simulink model "Stand_AOPO"  (R2018b)
settings: Solver=FixedStepAuto  StartTime=0.0  StopTime=inf  FixedStep=1e-3  RelTol=1e-3
libraries: simulink x17, simulink_extras x4, xpcutilitieslib x2, xpcrtudplib x2, opclib x1, sldrtlib x1
settings Model: Creator=YuORLOV  LastModifiedBy=9
settings DataIOCC: SaveTime=off
settings OptimizationCC: BlockReduction=off
settings DebuggingCC: LibraryContextMissingDiagnostic=none
settings SFSimCC: SimUseLocalCustomCode=off
settings RTWCC: RTWUseLocalCustomCode=off
settings CodeAppCC: StateflowObjectComments=on
settings SimscapeCC: SimscapeNormalizeSystem=off

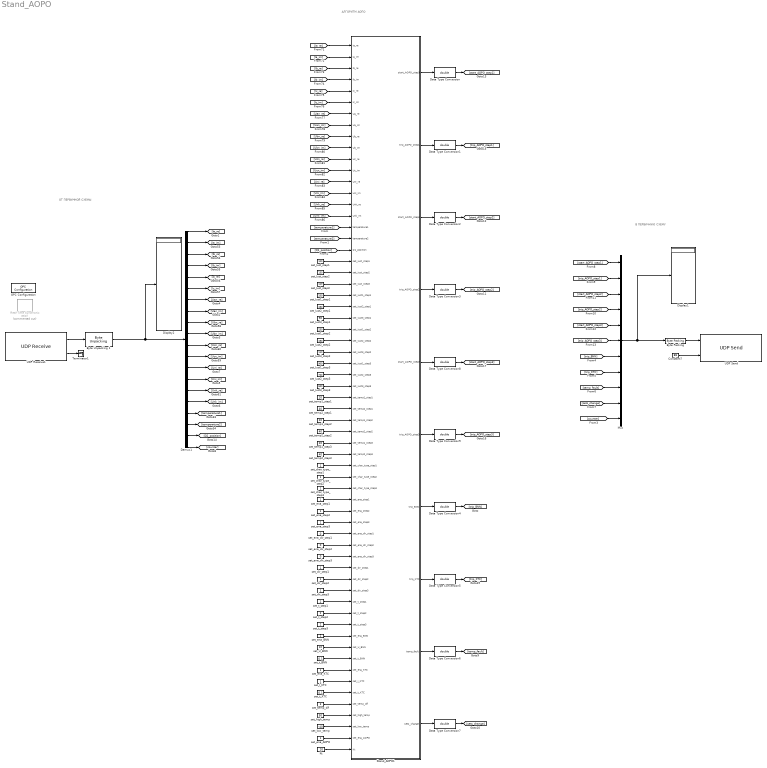
== system Stand_AOPO ==
  note: ОТ ПЕРВИЧНОЙ СХЕМЫ
  note: АЛГОРИТМ АОПО
  note: В ПЕРВИЧНУЮ СХЕМУ
  "Byte Packing " : xpcutilitieslib/Byte Packing   MaskPackedDataType=uint8  MaskUnpackedDataTypes={'double'}  MaskAlignment=1
  Byte Unpacking 1 : xpcutilitieslib/Byte Unpacking   MaskUnpackedDataTypes={'double'}  MaskUnpackedDataSizes={[20]}  MaskAlignment=1
      settings: SourceProductName=Simulink Real-Time  SourceProductBaseCode=XP
  Constant7 : Constant  Value=88
  Data Type Conversion{,1..9} (10 alike) : DataTypeConversion  OutDataTypeStr=double
  Demux1 : Demux  Outputs=20
  Display1 : Display
  Display2 : Display
  Kt : Constant  Value=20
  Mux : Mux  Inputs=11
  OPC Configuration : opclib/OPC Configuration  errMissingItems=Error  errReadWrite=Warn  errShutdown=Error  errRTViolation=Warn  rtEnable=on  speedup=1  showLatency=off  beingUsed=on
      settings: SourceProductName=OPC Toolbox  SourceProductBaseCode=OT
  Real-Time Synchronization : sldrtlib/Real-Time Synchronization  Commented=on  SampleTime=0.1  MaxMissedTicks=10  ShowMissedTicks=off  YieldWhenWaiting=off
  Stand_AOPO1 : Subsystem
  Terminator1 : Terminator
  UDP Receive1 : xpcrtudplib/UDP Receive  ipAddressVal=Use host-target connection  localPort=25001  rcvWidth=160  rcvFmAny=off  fmAddress=192.168.1.251  rcvMulticast=off  multicastAddress=[]  maxUDPQueue=8  sampleTime=1e-3
      settings: SourceProductName=Simulink Real-Time
  UDP Send : xpcrtudplib/UDP Send  ipAddressVal=Use host-target connection  localPort=25002  toAddress=192.168.1.251  toPort=8002  sampleTime=1e-3
      settings: SourceProductName=Simulink Real-Time  SourceProductBaseCode=XP
  set_I_KTC : Constant
  set_Iust1_step1 : Constant  Value=200
  set_Iust1_step2 : Constant  Value=250
  set_Iust1_step3 : Constant  Value=900
  set_Iust2_step1 : Constant  Value=160
  set_Iust2_step2 : Constant  Value=190
  set_Iust2_step3 : Constant  Value=700
  set_Iust3_step1 : Constant  Value=90
  set_Iust3_step2 : Constant  Value=110
  set_Iust3_step3 : Constant  Value=500
  set_Iust_step1 : Constant  Value=120
  set_Iust_step2 : Constant  Value=130
  set_Iust_step3 : Constant  Value=140
  set_U_BNN : Constant  Value=10
  set_char_type_step1 : Constant
  set_char_type_step2 : Constant
  set_char_type_step3 : Constant
  set_dir_step1 : Constant
  set_dir_step2 : Constant
  set_dir_step3 : Constant
  set_ena_AOPO : Constant
  set_ena_BNN : Constant
  set_ena_KTC : Constant
  set_ena_dir_step1 : Constant  Value=0
  set_ena_dir_step2 : Constant  Value=0
  set_ena_dir_step3 : Constant  Value=0
  set_ena_step1 : Constant
  set_ena_step2 : Constant
  set_ena_step3 : Constant
  set_high_temp : Constant  Value=50
  set_low_temp : Constant  Value=-40
  set_t_BNN : Constant  Value=0.1
  set_t_KTC : Constant  Value=0.1
  set_t_step1 : Constant  Value=2
  set_t_step2 : Constant  Value=2
  set_t_step3 : Constant  Value=2
  set_temp1_step1 : Constant  Value=20
  set_temp1_step2 : Constant  Value=20
  set_temp1_step3 : Constant  Value=20
  set_temp2_step1 : Constant  Value=40
  set_temp2_step2 : Constant  Value=40
  set_temp2_step3 : Constant  Value=40
  set_temp_dif : Constant  Value=3
  wires:
  Mux/1 -> Display1/1, "Byte Packing "/1
  Constant7/1 -> UDP Send/2
  "Byte Packing "/1 -> UDP Send/1
  set_Iust_step1/1 -> Stand_AOPO1/20(set_Iust_step1)
  set_Iust_step2/1 -> Stand_AOPO1/21(set_Iust_step2)
  set_U_BNN/1 -> Stand_AOPO1/54(set_U_BNN)
  set_t_step1/1 -> Stand_AOPO1/50(set_t_step1)
  set_t_step2/1 -> Stand_AOPO1/51(set_t_step2)
  set_t_BNN/1 -> Stand_AOPO1/55(set_t_BNN)
  set_I_KTC/1 -> Stand_AOPO1/57(set_I_KTC)
  set_t_KTC/1 -> Stand_AOPO1/58(set_t_KTC)
  set_ena_step1/1 -> Stand_AOPO1/41(set_ena_step1)
  set_ena_step2/1 -> Stand_AOPO1/42(set_ena_step2)
  set_ena_AOPO/1 -> Stand_AOPO1/62(set_ena_AOPO)
  set_ena_KTC/1 -> Stand_AOPO1/56(set_ena_KTC)
  set_dir_step2/1 -> Stand_AOPO1/48(set_dir_step2)
  set_dir_step1/1 -> Stand_AOPO1/47(set_dir_step1)
  set_ena_dir_step2/1 -> Stand_AOPO1/45(set_ena_dir_step2)
  set_ena_dir_step1/1 -> Stand_AOPO1/44(set_ena_dir_step1)
  set_ena_BNN/1 -> Stand_AOPO1/53(set_ena_BNN)
  set_char_type_step2/1 -> Stand_AOPO1/39(set_char_type_step2)
  set_char_type_step1/1 -> Stand_AOPO1/38(set_char_type_step1)
  set_temp2_step2/1 -> Stand_AOPO1/35(set_temp2_step2)
  set_temp1_step2/1 -> Stand_AOPO1/34(set_temp1_step2)
  set_temp2_step1/1 -> Stand_AOPO1/33(set_temp2_step1)
  set_temp1_step1/1 -> Stand_AOPO1/32(set_temp1_step1)
  set_Iust3_step2/1 -> Stand_AOPO1/28(set_Iust3_step2)
  set_Iust2_step2/1 -> Stand_AOPO1/27(set_Iust2_step2)
  set_Iust1_step2/1 -> Stand_AOPO1/26(set_Iust1_step2)
  set_Iust3_step1/1 -> Stand_AOPO1/25(set_Iust3_step1)
  set_Iust2_step1/1 -> Stand_AOPO1/24(set_Iust2_step1)
  set_Iust1_step1/1 -> Stand_AOPO1/23(set_Iust1_step1)
  Byte Unpacking 1/1 -> Demux1/1, Display2/1
  UDP Receive1/1 -> Byte Unpacking 1/1
  UDP Receive1/2 -> Terminator1/1
  Stand_AOPO1/1(start_AOPO_step1) -> Data Type Conversion/1
  Stand_AOPO1/2(trip_AOPO_step1) -> Data Type Conversion1/1
  Stand_AOPO1/3(start_AOPO_step2) -> Data Type Conversion2/1
  Stand_AOPO1/4(trip_AOPO_step2) -> Data Type Conversion3/1
  Stand_AOPO1/7(trip_BNN) -> Data Type Conversion4/1
  Stand_AOPO1/8(trip_KTC) -> Data Type Conversion5/1
  Kt/1 -> Stand_AOPO1/63(Kt)
  set_temp_dif/1 -> Stand_AOPO1/59(set_temp_dif)
  set_high_temp/1 -> Stand_AOPO1/60(set_high_temp)
  set_low_temp/1 -> Stand_AOPO1/61(set_low_temp)
  Stand_AOPO1/9(temp_fault) -> Data Type Conversion6/1
  Stand_AOPO1/10(sets_change) -> Data Type Conversion7/1
  Demux1/1 -> [Ia_re]
  Demux1/2 -> [Ia_im]
  Demux1/3 -> [Ib_re]
  Demux1/4 -> [Ib_im]
  Demux1/5 -> [Ic_re]
  Demux1/6 -> [Ic_im]
  [Ia_re] -> Stand_AOPO1/1(Ia_re)
  [Ia_im] -> Stand_AOPO1/2(Ia_im)
  [Ib_re] -> Stand_AOPO1/3(Ib_re)
  [Ib_im] -> Stand_AOPO1/4(Ib_im)
  [Ic_re] -> Stand_AOPO1/5(Ic_re)
  [Ic_im] -> Stand_AOPO1/6(Ic_im)
  Demux1/7 -> [Uan_re]
  Demux1/8 -> [Uan_im]
  Demux1/9 -> [Ubn_re]
  Demux1/10 -> [Ubn_im]
  Demux1/11 -> [Ucn_re]
  Demux1/12 -> [Ucn_im]
  Demux1/13 -> [Uni_re]
  Demux1/14 -> [Uni_im]
  Demux1/15 -> [Unk_re]
  Demux1/16 -> [Unk_im]
  Demux1/17 -> [temperature1]
  Demux1/18 -> [temperature2]
  Demux1/19 -> [Q1_position]
  [Uan_re] -> Stand_AOPO1/7(Ua_re)
  [Unk_im] -> Stand_AOPO1/16(Unk_im)
  [Unk_re] -> Stand_AOPO1/15(Unk_re)
  [Uni_im] -> Stand_AOPO1/14(Uni_im)
  [Uni_re] -> Stand_AOPO1/13(Uni_re)
  [Ucn_im] -> Stand_AOPO1/12(Uc_im)
  [Ucn_re] -> Stand_AOPO1/11(Uc_re)
  [Ubn_im] -> Stand_AOPO1/10(Ub_im)
  [Ubn_re] -> Stand_AOPO1/9(Ub_re)
  [Uan_im] -> Stand_AOPO1/8(Ua_im)
  [temperature1] -> Stand_AOPO1/17(temperature1)
  [temperature2] -> Stand_AOPO1/18(temperature2)
  [Q1_position] -> Stand_AOPO1/19(Q1_position)
  Demux1/20 -> [counter]
  Data Type Conversion4/1 -> [trip_BNN]
  Data Type Conversion5/1 -> [trip_KTC]
  Data Type Conversion6/1 -> [temp_fault]
  Data Type Conversion7/1 -> [sets_change]
  Data Type Conversion3/1 -> [trip_AOPO_step2]
  Data Type Conversion2/1 -> [start_AOPO_step2]
  Data Type Conversion/1 -> [start_AOPO_step1]
  Data Type Conversion1/1 -> [trip_AOPO_step1]
  [trip_AOPO_step1] -> Mux/2
  [start_AOPO_step1] -> Mux/1
  [start_AOPO_step2] -> Mux/3
  [trip_AOPO_step2] -> Mux/4
  Data Type Conversion8/1 -> [start_AOPO_step3]
  Data Type Conversion9/1 -> [trip_AOPO_step3]
  Stand_AOPO1/6(trip_AOPO_step3) -> Data Type Conversion9/1
  Stand_AOPO1/5(start_AOPO_step3) -> Data Type Conversion8/1
  [trip_BNN] -> Mux/7
  [trip_KTC] -> Mux/8
  [temp_fault] -> Mux/9
  [sets_change] -> Mux/10
  [counter] -> Mux/11
  [start_AOPO_step3] -> Mux/5
  [trip_AOPO_step3] -> Mux/6
  set_t_step3/1 -> Stand_AOPO1/52(set_t_step3)
  set_dir_step3/1 -> Stand_AOPO1/49(set_dir_step3)
  set_ena_dir_step3/1 -> Stand_AOPO1/46(set_ena_dir_step3)
  set_ena_step3/1 -> Stand_AOPO1/43(set_ena_step3)
  set_char_type_step3/1 -> Stand_AOPO1/40(set_char_type_step3)
  set_temp1_step3/1 -> Stand_AOPO1/36(set_temp1_step3)
  set_temp2_step3/1 -> Stand_AOPO1/37(set_temp2_step3)
  set_Iust2_step3/1 -> Stand_AOPO1/30(set_Iust2_step3)
  set_Iust1_step3/1 -> Stand_AOPO1/29(set_Iust1_step3)
  set_Iust3_step3/1 -> Stand_AOPO1/31(set_Iust3_step3)
  set_Iust_step3/1 -> Stand_AOPO1/22(set_Iust_step3)

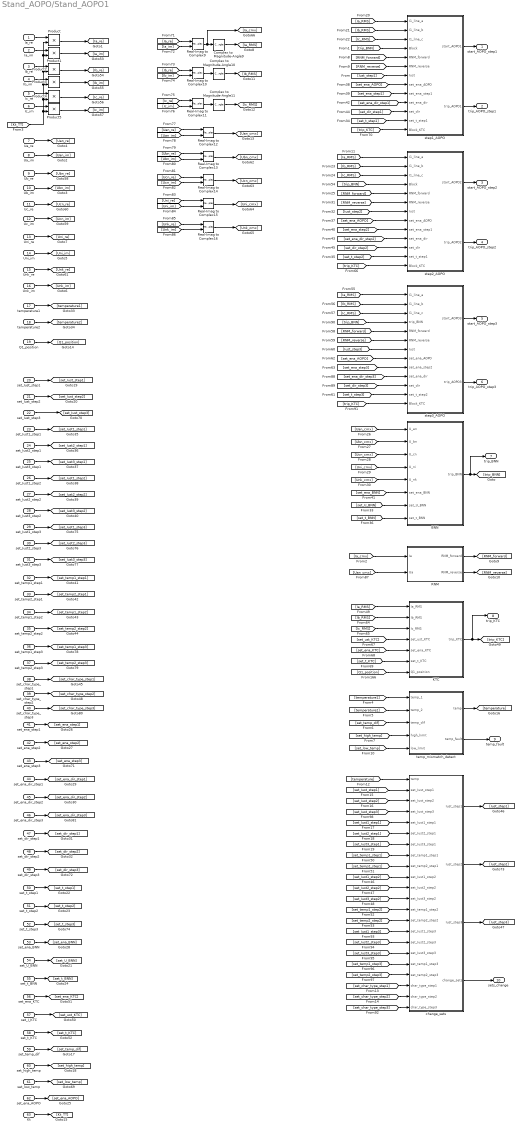
== system Stand_AOPO/Stand_AOPO1 ==
  Ia_re : Inport
  Ia_im : Inport  Port=2
  Ib_re : Inport  Port=3
  Ib_im : Inport  Port=4
  Ic_re : Inport  Port=5
  Ic_im : Inport  Port=6
  Ua_re : Inport  Port=7
  Ua_im : Inport  Port=8
  Ub_re : Inport  Port=9
  Ub_im : Inport  Port=10
  Uc_re : Inport  Port=11
  Uc_im : Inport  Port=12
  Uni_re : Inport  Port=13
  Uni_im : Inport  Port=14
  Unk_re : Inport  Port=15
  Unk_im : Inport  Port=16
  temperature1 : Inport  Port=17
  temperature2 : Inport  Port=18
  Q1_position : Inport  Port=19
  set_Iust_step1 : Inport  Port=20
  set_Iust_step2 : Inport  Port=21
  set_Iust_step3 : Inport  Port=22
  set_Iust1_step1 : Inport  Port=23
  set_Iust2_step1 : Inport  Port=24
  set_Iust3_step1 : Inport  Port=25
  set_Iust1_step2 : Inport  Port=26
  set_Iust2_step2 : Inport  Port=27
  set_Iust3_step2 : Inport  Port=28
  set_Iust1_step3 : Inport  Port=29
  set_Iust2_step3 : Inport  Port=30
  set_Iust3_step3 : Inport  Port=31
  set_temp1_step1 : Inport  Port=32
  set_temp2_step1 : Inport  Port=33
  set_temp1_step2 : Inport  Port=34
  set_temp2_step2 : Inport  Port=35
  set_temp1_step3 : Inport  Port=36
  set_temp2_step3 : Inport  Port=37
  set_char_type_step1 : Inport  Port=38
  set_char_type_step2 : Inport  Port=39
  set_char_type_step3 : Inport  Port=40
  set_ena_step1 : Inport  Port=41
  set_ena_step2 : Inport  Port=42
  set_ena_step3 : Inport  Port=43
  set_ena_dir_step1 : Inport  Port=44
  set_ena_dir_step2 : Inport  Port=45
  set_ena_dir_step3 : Inport  Port=46
  set_dir_step1 : Inport  Port=47
  set_dir_step2 : Inport  Port=48
  set_dir_step3 : Inport  Port=49
  set_t_step1 : Inport  Port=50
  set_t_step2 : Inport  Port=51
  set_t_step3 : Inport  Port=52
  set_ena_BNN : Inport  Port=53
  set_U_BNN : Inport  Port=54
  set_t_BNN : Inport  Port=55
  set_ena_KTC : Inport  Port=56
  set_I_KTC : Inport  Port=57
  set_t_KTC : Inport  Port=58
  set_temp_dif : Inport  Port=59
  set_high_temp : Inport  Port=60
  set_low_temp : Inport  Port=61
  set_ena_AOPO : Inport  Port=62
  Kt : Inport  Port=63
  BNN : Subsystem
  Complex to Magnitude-Angle10 : ComplexToMagnitudeAngle  Output=Magnitude
  Complex to Magnitude-Angle11 : ComplexToMagnitudeAngle  Output=Magnitude
  Complex to Magnitude-Angle9 : ComplexToMagnitudeAngle  Output=Magnitude
  KTC : Subsystem
  Product{,1..5} (6 alike) : Product
  RNM : Subsystem
  Real-Imag to Complex{9..16} (8 alike) : RealImagToComplex
  change_sets : Subsystem
  step1_AOPO : Subsystem
  step2_AOPO : Subsystem
  step3_AOPO : Subsystem
  temp_mismatch_detect : Subsystem
  start_AOPO_step1 : Outport
  trip_AOPO_step1 : Outport  Port=2
  start_AOPO_step2 : Outport  Port=3
  trip_AOPO_step2 : Outport  Port=4
  start_AOPO_step3 : Outport  Port=5
  trip_AOPO_step3 : Outport  Port=6
  trip_BNN : Outport  Port=7
  trip_KTC : Outport  Port=8
  temp_fault : Outport  Port=9
  sets_change : Outport  Port=10
  wires:
  RNM/1(RNM_forward) -> [RNM_forward]
  RNM/2(RNM_reverse) -> [RNM_reverse]
  [Ucn_cmx] -> BNN/3(U_cn)
  [Ubn_cmx] -> BNN/2(U_bn)
  [Unk_cmx] -> BNN/5(U_nk)
  [Uan_cmx] -> BNN/1(U_an)
  [Uni_cmx] -> BNN/4(U_ni)
  [Ic_RMS] -> step1_AOPO/3(I1_line_c)
  [Ib_RMS] -> step1_AOPO/2(I1_line_b)
  [RNM_forward] -> step1_AOPO/5(RNM_forward)
  [RNM_reverse] -> step1_AOPO/6(RNM_reverse)
  [trip_BNN] -> step1_AOPO/4(Block)
  BNN/1(trip_BNN) -> trip_BNN/1, [trip_BNN]
  [Ia_RMS] -> step1_AOPO/1(I1_line_a)
  step1_AOPO/2(trip_AOPO1) -> trip_AOPO_step1/1
  [Ia_cmx] -> RNM/1(Ia)
  Ua_re/1 -> [Uan_re]
  step1_AOPO/1(start_AOPO1) -> start_AOPO_step1/1
  Uni_re/1 -> [Uni_re]
  step2_AOPO/1(start_AOPO2) -> start_AOPO_step2/1
  step2_AOPO/2(trip_AOPO2) -> trip_AOPO_step2/1
  [Ia_RMS] -> step2_AOPO/1(I1_line_a)
  [RNM_reverse] -> step2_AOPO/6(RNM_reverse)
  [RNM_forward] -> step2_AOPO/5(RNM_forward)
  [Ib_RMS] -> step2_AOPO/2(I1_line_b)
  [Ic_RMS] -> step2_AOPO/3(I1_line_c)
  set_Iust_step1/1 -> [set_Iust_step1]
  set_Iust_step2/1 -> [set_Iust_step2]
  set_U_BNN/1 -> [set_U_BNN]
  set_t_step1/1 -> [set_t_step1]
  set_t_step2/1 -> [set_t_step2]
  set_t_BNN/1 -> [set_t_BNN]
  [set_t_BNN] -> BNN/8(set_t_BNN)
  [set_t_step1] -> step1_AOPO/12(set_t_step1)
  [set_U_BNN] -> BNN/7(set_U_BNN)
  set_ena_AOPO/1 -> [set_ena_AOPO]
  set_ena_step1/1 -> [set_ena_step1]
  set_ena_step2/1 -> [set_ena_step2]
  set_ena_BNN/1 -> [set_ena_BNN]
  [set_ena_AOPO] -> step1_AOPO/8(set_ena_AOPO)
  [set_ena_BNN] -> BNN/6(set_ena_BNN)
  [set_ena_step1] -> step1_AOPO/9(set_ena_step1)
  set_ena_dir_step1/1 -> [set_ena_dir_step1]
  set_ena_dir_step2/1 -> [set_ena_dir_step2]
  [set_ena_dir_step1] -> step1_AOPO/10(set_ena_dir)
  set_dir_step2/1 -> [set_dir_step2]
  set_dir_step1/1 -> [set_dir_step1]
  [set_dir_step1] -> step1_AOPO/11(set_dir)
  temperature1/1 -> [temperature1]
  temperature2/1 -> [temperature2]
  set_Iust2_step1/1 -> [set_Iust2_step1]
  set_Iust1_step1/1 -> [set_Iust1_step1]
  set_Iust3_step1/1 -> [set_Iust3_step1]
  set_Iust3_step2/1 -> [set_Iust3_step2]
  set_Iust1_step2/1 -> [set_Iust1_step2]
  set_Iust2_step2/1 -> [set_Iust2_step2]
  set_temp1_step1/1 -> [set_temp1_step1]
  set_temp2_step1/1 -> [set_temp2_step1]
  set_temp2_step2/1 -> [set_temp2_step2]
  set_temp1_step2/1 -> [set_temp1_step2]
  set_char_type_step1/1 -> [set_char_type_step1]
  [Iust_step1] -> step1_AOPO/7(Iust)
  set_char_type_step2/1 -> [set_char_type_step2]
  [Ia_RMS] -> KTC/1(Ia_RMS)
  [Ib_RMS] -> KTC/2(Ib_RMS)
  [Ic_RMS] -> KTC/3(Ic_RMS)
  [set_ust_KTC] -> KTC/4(set_ust_KTC)
  KTC/1(trip_KTC) -> trip_KTC/1, [trip_KTC]
  [set_ena_KTC] -> KTC/5(set_ena_KTC)
  [set_t_KTC] -> KTC/6(set_t_KTC)
  set_I_KTC/1 -> [set_ust_KTC]
  set_ena_KTC/1 -> [set_ena_KTC]
  set_t_KTC/1 -> [set_t_KTC]
  [trip_KTC] -> step1_AOPO/13(Block_KTC)
  Real-Imag to Complex9/1 -> [Ia_cmx], Complex to Magnitude-Angle9/1
  [Ia_re] -> Real-Imag to Complex9/1
  [Ia_im] -> Real-Imag to Complex9/2
  Real-Imag to Complex10/1 -> Complex to Magnitude-Angle10/1
  Real-Imag to Complex11/1 -> Complex to Magnitude-Angle11/1
  [Ib_re] -> Real-Imag to Complex10/1
  [Ib_im] -> Real-Imag to Complex10/2
  [Ic_re] -> Real-Imag to Complex11/1
  [Ic_im] -> Real-Imag to Complex11/2
  Ua_im/1 -> [Uan_im]
  Ub_im/1 -> [Ubn_im]
  Ub_re/1 -> [Ubn_re]
  Uc_re/1 -> [Ucn_re]
  Uc_im/1 -> [Ucn_im]
  Real-Imag to Complex12/1 -> [Uan_cmx]
  [Uan_re] -> Real-Imag to Complex12/1
  [Uan_im] -> Real-Imag to Complex12/2
  Real-Imag to Complex13/1 -> [Ubn_cmx]
  [Ubn_re] -> Real-Imag to Complex13/1
  [Ubn_im] -> Real-Imag to Complex13/2
  Real-Imag to Complex14/1 -> [Ucn_cmx]
  [Ucn_re] -> Real-Imag to Complex14/1
  [Ucn_im] -> Real-Imag to Complex14/2
  Uni_im/1 -> [Uni_im]
  Unk_im/1 -> [Unk_im]
  Unk_re/1 -> [Unk_re]
  Real-Imag to Complex16/1 -> [Unk_cmx]
  Real-Imag to Complex15/1 -> [Uni_cmx]
  [Uni_re] -> Real-Imag to Complex15/1
  [Uni_im] -> Real-Imag to Complex15/2
  [Unk_re] -> Real-Imag to Complex16/1
  [Unk_im] -> Real-Imag to Complex16/2
  Complex to Magnitude-Angle11/1 -> [Ic_RMS]
  Complex to Magnitude-Angle10/1 -> [Ib_RMS]
  Complex to Magnitude-Angle9/1 -> [Ia_RMS]
  [Uan_cmx] -> RNM/2(Ua)
  [Q1_position] -> KTC/7(Q1_position)
  Q1_position/1 -> [Q1_position]
  Kt/1 -> [Kt_TT]
  Ia_re/1 -> Product/1
  Product/1 -> [Ia_re]
  Ia_im/1 -> Product1/1
  Product1/1 -> [Ia_im]
  Ib_re/1 -> Product2/1
  Product2/1 -> [Ib_re]
  Ib_im/1 -> Product3/1
  Product3/1 -> [Ib_im]
  Ic_re/1 -> Product4/1
  Ic_im/1 -> Product5/1
  [Kt_TT] -> Product5/2, Product4/2, Product3/2, Product2/2, Product1/2, Product/2
  Product4/1 -> [Ic_re]
  Product5/1 -> [Ic_im]
  [temperature1] -> temp_mismatch_detect/1(temp_1)
  [temperature2] -> temp_mismatch_detect/2(temp_2)
  [set_temp_dif] -> temp_mismatch_detect/3(temp_dif)
  [set_high_temp] -> temp_mismatch_detect/4(high_limit)
  [set_low_temp] -> temp_mismatch_detect/5(low_limit)
  temp_mismatch_detect/1(temp) -> [temperature]
  set_temp_dif/1 -> [set_temp_dif]
  set_high_temp/1 -> [set_high_temp]
  set_low_temp/1 -> [set_low_temp]
  change_sets/1(Iust_step1) -> [Iust_step1]
  change_sets/3(Iust_step3) -> [Iust_step3]
  [temperature] -> change_sets/1(temp)
  [set_char_type_step2] -> change_sets/21(char_type_step2)
  [set_char_type_step1] -> change_sets/20(char_type_step1)
  [set_Iust_step1] -> change_sets/2(set_Iust_step1)
  [set_Iust_step2] -> change_sets/3(set_Iust_step2)
  [set_Iust1_step1] -> change_sets/5(set_Iust1_step1)
  [set_Iust2_step1] -> change_sets/6(set_Iust2_step1)
  [set_Iust3_step1] -> change_sets/7(set_Iust3_step1)
  [set_Iust1_step2] -> change_sets/10(set_Iust1_step2)
  [set_Iust2_step2] -> change_sets/11(set_Iust2_step2)
  [set_Iust3_step2] -> change_sets/12(set_Iust3_step2)
  [set_temp1_step1] -> change_sets/8(set_temp1_step1)
  [set_temp2_step1] -> change_sets/9(set_temp2_step1)
  [set_temp1_step2] -> change_sets/13(set_temp1_step2)
  [set_temp2_step2] -> change_sets/14(set_temp2_step2)
  temp_mismatch_detect/2(temp_fault) -> temp_fault/1
  change_sets/4(change_sets) -> sets_change/1
  [trip_BNN] -> step2_AOPO/4(Block)
  [trip_BNN] -> step3_AOPO/4(trip_BNN)
  [Ic_RMS] -> step3_AOPO/3(I1_line_c)
  [Ib_RMS] -> step3_AOPO/2(I1_line_b)
  [RNM_forward] -> step3_AOPO/5(RNM_forward)
  [RNM_reverse] -> step3_AOPO/6(RNM_reverse)
  [Ia_RMS] -> step3_AOPO/1(I1_line_a)
  step3_AOPO/2(trip_AOPO3) -> trip_AOPO_step3/1
  step3_AOPO/1(start_AOPO3) -> start_AOPO_step3/1
  [set_ena_dir_step3] -> step3_AOPO/10(set_ena_dir)
  [set_ena_step3] -> step3_AOPO/9(set_ena_step2)
  [set_dir_step3] -> step3_AOPO/11(set_dir)
  [set_ena_AOPO] -> step3_AOPO/8(set_ena_AOPO)
  [set_t_step3] -> step3_AOPO/12(set_t_step2)
  [Iust_step3] -> step3_AOPO/7(Iust)
  [trip_KTC] -> step3_AOPO/13(Block_KTC)
  [set_ena_dir_step2] -> step2_AOPO/10(set_ena_dir)
  [set_ena_step2] -> step2_AOPO/9(set_ena_step1)
  [set_dir_step2] -> step2_AOPO/11(set_dir)
  [set_ena_AOPO] -> step2_AOPO/8(set_ena_AOPO)
  [set_t_step2] -> step2_AOPO/12(set_t_step1)
  [Iust_step2] -> step2_AOPO/7(Iust)
  [trip_KTC] -> step2_AOPO/13(Block_KTC)
  [set_Iust1_step3] -> change_sets/15(set_Iust1_step3)
  [set_Iust2_step3] -> change_sets/16(set_Iust2_step3)
  [set_Iust3_step3] -> change_sets/17(set_Iust3_step3)
  [set_temp1_step3] -> change_sets/18(set_temp1_step3)
  [set_temp2_step3] -> change_sets/19(set_temp2_step3)
  [set_char_type_step3] -> change_sets/22(char_type_step3)
  [set_Iust_step3] -> change_sets/4(set_Iust_step3)
  change_sets/2(Iust_step2) -> [Iust_step2]
  set_Iust_step3/1 -> [set_Iust_step3]
  set_Iust1_step3/1 -> [set_Iust1_step3]
  set_Iust2_step3/1 -> [set_Iust2_step3]
  set_Iust3_step3/1 -> [set_Iust3_step3]
  set_temp1_step3/1 -> [set_temp1_step3]
  set_temp2_step3/1 -> [set_temp2_step3]
  set_char_type_step3/1 -> [set_char_type_step3]
  set_ena_step3/1 -> [set_ena_step3]
  set_ena_dir_step3/1 -> [set_ena_dir_step3]
  set_dir_step3/1 -> [set_dir_step3]
  set_t_step3/1 -> [set_t_step3]

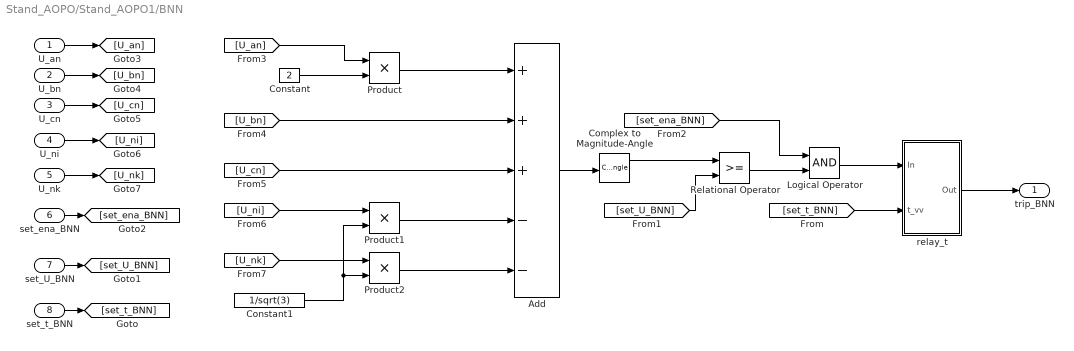
== system Stand_AOPO/Stand_AOPO1/BNN ==
  U_an : Inport
  U_bn : Inport  Port=2
  U_cn : Inport  Port=3
  U_ni : Inport  Port=4
  U_nk : Inport  Port=5
  set_ena_BNN : Inport  Port=6
  set_U_BNN : Inport  Port=7
  set_t_BNN : Inport  Port=8
  Add : Sum  Inputs=+++--
  Complex to Magnitude-Angle : ComplexToMagnitudeAngle
  Constant : Constant  Value=2
  Constant1 : Constant  Value=1/sqrt(3)
  Logical Operator : Logic  AllPortsSameDT=off  OutDataTypeStr=boolean
  Product : Product
  Product1 : Product
  Product2 : Product
  Relational Operator : RelationalOperator  OutDataTypeStr=boolean  RndMeth=Simplest
  relay_t : Subsystem
  trip_BNN : Outport
  wires:
  Product1/1 -> Add/4
  Constant1/1 -> Product1/2, Product2/2
  Product2/1 -> Add/5
  Constant/1 -> Product/2
  Product/1 -> Add/1
  [set_U_BNN] -> Relational Operator/2
  relay_t/1(Out) -> trip_BNN/1
  set_t_BNN/1 -> [set_t_BNN]
  set_U_BNN/1 -> [set_U_BNN]
  set_ena_BNN/1 -> [set_ena_BNN]
  U_an/1 -> [U_an]
  U_bn/1 -> [U_bn]
  U_cn/1 -> [U_cn]
  U_ni/1 -> [U_ni]
  U_nk/1 -> [U_nk]
  [U_an] -> Product/1
  [U_bn] -> Add/2
  [U_cn] -> Add/3
  [U_ni] -> Product1/1
  [U_nk] -> Product2/1
  Relational Operator/1 -> Logical Operator/2
  Logical Operator/1 -> relay_t/1(In)
  [set_ena_BNN] -> Logical Operator/1
  Complex to Magnitude-Angle/1 -> Relational Operator/1
  Add/1 -> Complex to Magnitude-Angle/1
  [set_t_BNN] -> relay_t/2(t_vv)

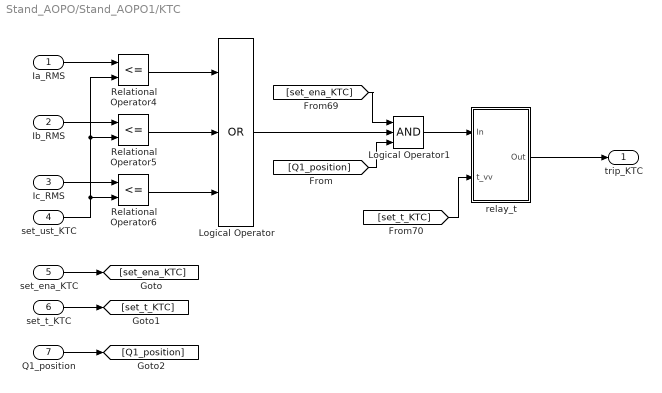
== system Stand_AOPO/Stand_AOPO1/KTC ==
  Ia_RMS : Inport
  Ib_RMS : Inport  Port=2
  Ic_RMS : Inport  Port=3
  set_ust_KTC : Inport  Port=4
  set_ena_KTC : Inport  Port=5
  set_t_KTC : Inport  Port=6
  Q1_position : Inport  Port=7
  Logical Operator : Logic  Operator=OR  Inputs=3  AllPortsSameDT=off  OutDataTypeStr=boolean
  Logical Operator1 : Logic  Inputs=3  AllPortsSameDT=off  OutDataTypeStr=boolean
  Relational Operator4 : RelationalOperator  Operator=<=  OutDataTypeStr=boolean  RndMeth=Simplest
  Relational Operator5 : RelationalOperator  Operator=<=  OutDataTypeStr=boolean  RndMeth=Simplest
  Relational Operator6 : RelationalOperator  Operator=<=  OutDataTypeStr=boolean  RndMeth=Simplest
  relay_t : Subsystem
  trip_KTC : Outport
  wires:
  set_ust_KTC/1 -> Relational Operator4/2, Relational Operator5/2, Relational Operator6/2
  [set_ena_KTC] -> Logical Operator1/1
  Relational Operator6/1 -> Logical Operator/3
  Ia_RMS/1 -> Relational Operator4/1
  Logical Operator/1 -> Logical Operator1/2
  [set_t_KTC] -> relay_t/2(t_vv)
  Relational Operator4/1 -> Logical Operator/1
  Relational Operator5/1 -> Logical Operator/2
  Logical Operator1/1 -> relay_t/1(In)
  Ic_RMS/1 -> Relational Operator6/1
  Ib_RMS/1 -> Relational Operator5/1
  relay_t/1(Out) -> trip_KTC/1
  set_ena_KTC/1 -> [set_ena_KTC]
  set_t_KTC/1 -> [set_t_KTC]
  Q1_position/1 -> [Q1_position]
  [Q1_position] -> Logical Operator1/3

== system Stand_AOPO/Stand_AOPO1/RNM ==
  Ia : Inport
  Ua : Inport  Port=2
  Abs : Abs
  Compare To Constant : simulink/Logic and Bit Operations/Compare To Constant  relop=<=  const=0.5*pi  OutDataTypeStr=boolean
  Complex to Magnitude-Angle : ComplexToMagnitudeAngle
  Divide : Product  Inputs=/*
  Logical Operator : Logic  Operator=NOT  AllPortsSameDT=off  OutDataTypeStr=boolean
  RNM_forward : Outport
  RNM_reverse : Outport  Port=2
  wires:
  Compare To Constant/1 -> Logical Operator/1, RNM_forward/1
  Logical Operator/1 -> RNM_reverse/1
  Ia/1 -> Divide/1
  Ua/1 -> Divide/2
  Abs/1 -> Compare To Constant/1
  Divide/1 -> Complex to Magnitude-Angle/1
  Complex to Magnitude-Angle/2 -> Abs/1

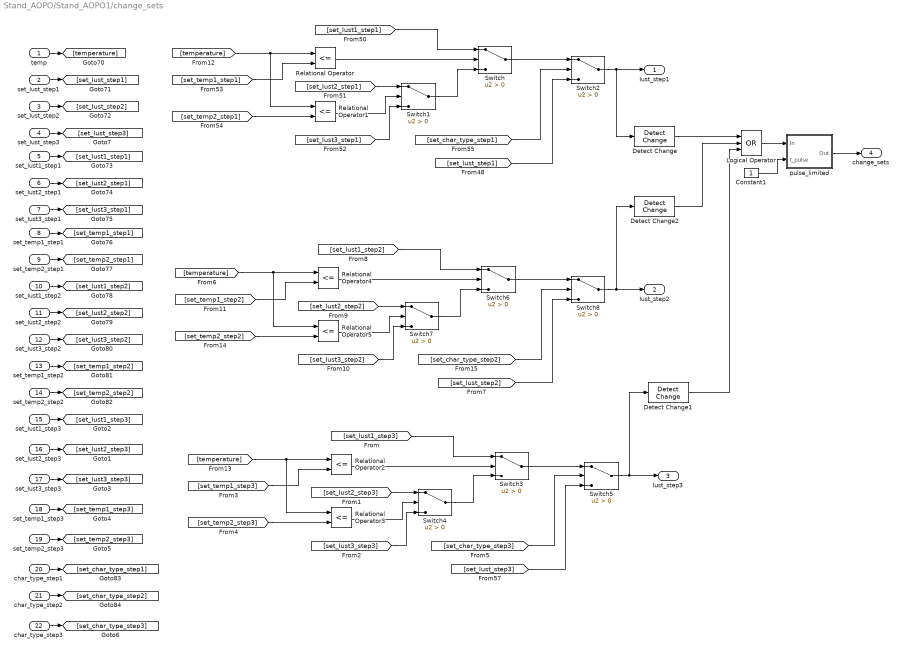
== system Stand_AOPO/Stand_AOPO1/change_sets ==
  temp : Inport
  set_Iust_step1 : Inport  Port=2
  set_Iust_step2 : Inport  Port=3
  set_Iust_step3 : Inport  Port=4
  set_Iust1_step1 : Inport  Port=5
  set_Iust2_step1 : Inport  Port=6
  set_Iust3_step1 : Inport  Port=7
  set_temp1_step1 : Inport  Port=8
  set_temp2_step1 : Inport  Port=9
  set_Iust1_step2 : Inport  Port=10
  set_Iust2_step2 : Inport  Port=11
  set_Iust3_step2 : Inport  Port=12
  set_temp1_step2 : Inport  Port=13
  set_temp2_step2 : Inport  Port=14
  set_Iust1_step3 : Inport  Port=15
  set_Iust2_step3 : Inport  Port=16
  set_Iust3_step3 : Inport  Port=17
  set_temp1_step3 : Inport  Port=18
  set_temp2_step3 : Inport  Port=19
  char_type_step1 : Inport  Port=20
  char_type_step2 : Inport  Port=21
  char_type_step3 : Inport  Port=22
  Constant1 : Constant
  Detect Change : simulink/Logic and Bit Operations/Detect Change  vinit=0  OutDataTypeStr=boolean
  Detect Change1 : simulink/Logic and Bit Operations/Detect Change  vinit=0  OutDataTypeStr=boolean
  Detect Change2 : simulink/Logic and Bit Operations/Detect Change  vinit=0  OutDataTypeStr=boolean
  Logical Operator : Logic  Operator=OR  Inputs=3  AllPortsSameDT=off  OutDataTypeStr=boolean
  Relational Operator{,1..5} (6 alike) : RelationalOperator  Operator=<=  OutDataTypeStr=boolean  RndMeth=Simplest
  Switch{,1..8} (9 alike) : Switch  Criteria=u2 > Threshold
  pulse_limited : Subsystem
  Iust_step1 : Outport
  Iust_step2 : Outport  Port=2
  Iust_step3 : Outport  Port=3
  change_sets : Outport  Port=4
  wires:
  [set_char_type_step1] -> Switch2/2
  [set_temp2_step3] -> Relational Operator3/2
  set_Iust2_step1/1 -> [set_Iust2_step1]
  set_Iust3_step2/1 -> [set_Iust3_step2]
  [set_temp1_step1] -> Relational Operator/2
  [set_temp2_step1] -> Relational Operator1/2
  temp/1 -> [temperature]
  set_Iust_step2/1 -> [set_Iust_step2]
  Switch5/1 -> Detect Change1/1, Iust_step3/1
  [set_Iust1_step3] -> Switch3/1
  [set_Iust3_step1] -> Switch1/3
  [set_Iust_step1] -> Switch2/3
  [set_Iust3_step3] -> Switch4/3
  char_type_step2/1 -> [set_char_type_step2]
  [set_Iust_step3] -> Switch5/3
  [set_temp1_step3] -> Relational Operator2/2
  [set_Iust2_step1] -> Switch1/1
  set_Iust_step1/1 -> [set_Iust_step1]
  [temperature] -> Relational Operator2/1, Relational Operator3/1
  char_type_step1/1 -> [set_char_type_step1]
  [set_Iust2_step3] -> Switch4/1
  Switch4/1 -> Switch3/3
  set_Iust1_step1/1 -> [set_Iust1_step1]
  Relational Operator1/1 -> Switch1/2
  Relational Operator2/1 -> Switch3/2
  Switch1/1 -> Switch/3
  Switch/1 -> Switch2/1
  Relational Operator/1 -> Switch/2
  [set_char_type_step3] -> Switch5/2
  Switch3/1 -> Switch5/1
  [temperature] -> Relational Operator1/1, Relational Operator/1
  [set_Iust1_step1] -> Switch/1
  set_Iust1_step2/1 -> [set_Iust1_step2]
  Relational Operator3/1 -> Switch4/2
  Switch2/1 -> Detect Change/1, Iust_step1/1
  set_temp2_step2/1 -> [set_temp2_step2]
  set_temp2_step1/1 -> [set_temp2_step1]
  set_temp1_step1/1 -> [set_temp1_step1]
  set_Iust3_step1/1 -> [set_Iust3_step1]
  set_Iust2_step2/1 -> [set_Iust2_step2]
  set_temp1_step2/1 -> [set_temp1_step2]
  Detect Change/1 -> Logical Operator/1
  Detect Change1/1 -> Logical Operator/3
  Logical Operator/1 -> pulse_limited/1(In)
  pulse_limited/1(Out) -> change_sets/1
  Constant1/1 -> pulse_limited/2(t_pulse)
  set_Iust1_step3/1 -> [set_Iust1_step3]
  set_Iust2_step3/1 -> [set_Iust2_step3]
  set_Iust3_step3/1 -> [set_Iust3_step3]
  set_temp1_step3/1 -> [set_temp1_step3]
  set_temp2_step3/1 -> [set_temp2_step3]
  char_type_step3/1 -> [set_char_type_step3]
  Relational Operator5/1 -> Switch7/2
  Switch6/1 -> Switch8/1
  [set_char_type_step2] -> Switch8/2
  Relational Operator4/1 -> Switch6/2
  Switch7/1 -> Switch6/3
  [set_Iust2_step2] -> Switch7/1
  [temperature] -> Relational Operator5/1, Relational Operator4/1
  [set_temp1_step2] -> Relational Operator4/2
  [set_Iust_step2] -> Switch8/3
  [set_Iust3_step2] -> Switch7/3
  [set_Iust1_step2] -> Switch6/1
  Switch8/1 -> Iust_step2/1, Detect Change2/1
  [set_temp2_step2] -> Relational Operator5/2
  Detect Change2/1 -> Logical Operator/2
  set_Iust_step3/1 -> [set_Iust_step3]

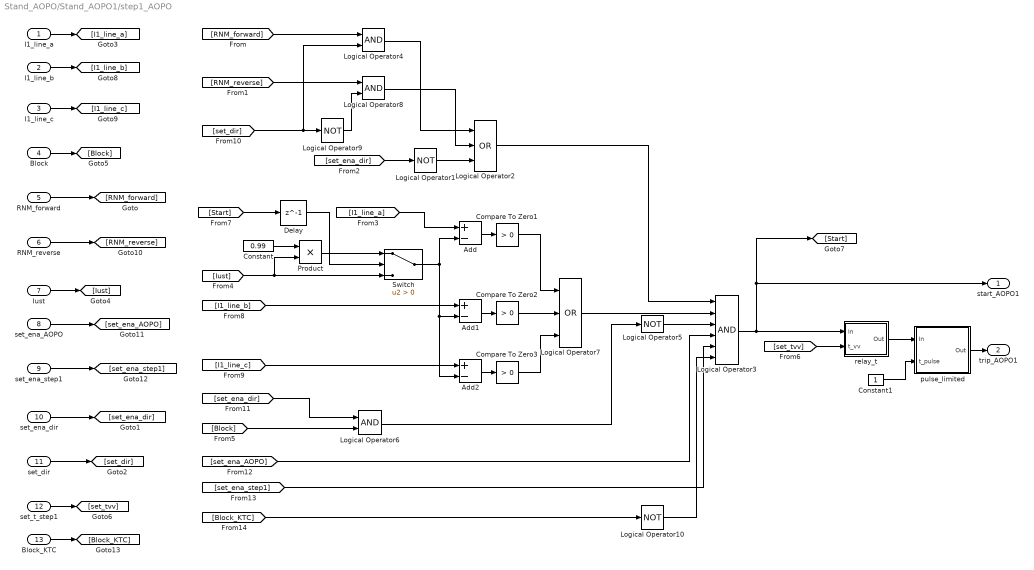
== system Stand_AOPO/Stand_AOPO1/step1_AOPO ==
  I1_line_a : Inport
  I1_line_b : Inport  Port=2
  I1_line_c : Inport  Port=3
  Block : Inport  Port=4
  RNM_forward : Inport  Port=5
  RNM_reverse : Inport  Port=6
  Iust : Inport  Port=7
  set_ena_AOPO : Inport  Port=8
  set_ena_step1 : Inport  Port=9
  set_ena_dir : Inport  Port=10
  set_dir : Inport  Port=11
  set_t_step1 : Inport  Port=12
  Block_KTC : Inport  Port=13
  Add : Sum  Inputs=+-
  Add1 : Sum  Inputs=+-
  Add2 : Sum  Inputs=+-
  Compare To Zero1 : simulink/Logic and Bit Operations/Compare To Zero  relop=>  OutDataTypeStr=boolean
  Compare To Zero2 : simulink/Logic and Bit Operations/Compare To Zero  relop=>  OutDataTypeStr=boolean
  Compare To Zero3 : simulink/Logic and Bit Operations/Compare To Zero  relop=>  OutDataTypeStr=boolean
  Constant : Constant  Value=0.99
  Constant1 : Constant
  Delay : Delay  DelayLength=1  InitialCondition=0
  Logical Operator{1,5,9..10} (4 alike) : Logic  Operator=NOT  AllPortsSameDT=off  OutDataTypeStr=boolean
  Logical Operator2 : Logic  Operator=OR  Inputs=3  AllPortsSameDT=off  OutDataTypeStr=boolean
  Logical Operator3 : Logic  Inputs=6  AllPortsSameDT=off  OutDataTypeStr=boolean
  Logical Operator4 : Logic  AllPortsSameDT=off  OutDataTypeStr=boolean
  Logical Operator6 : Logic  AllPortsSameDT=off  OutDataTypeStr=boolean
  Logical Operator7 : Logic  Operator=OR  Inputs=3  AllPortsSameDT=off  OutDataTypeStr=boolean
  Logical Operator8 : Logic  AllPortsSameDT=off  OutDataTypeStr=boolean
  Product : Product
  Switch : Switch  Criteria=u2 > Threshold
  pulse_limited : Subsystem
  relay_t : Subsystem
  start_AOPO1 : Outport
  trip_AOPO1 : Outport  Port=2
  wires:
  I1_line_a/1 -> [I1_line_a]
  Logical Operator5/1 -> Logical Operator3/3
  set_t_step1/1 -> [set_tvv]
  Iust/1 -> [Iust]
  Block/1 -> [Block]
  Add/1 -> Compare To Zero1/1
  [I1_line_a] -> Add/1
  [Iust] -> Switch/3, Product/2
  Constant/1 -> Product/1
  Product/1 -> Switch/1
  Switch/1 -> Add2/2, Add1/2, Add/2
  [Start] -> Delay/1
  Delay/1 -> Switch/2
  I1_line_c/1 -> [I1_line_c]
  I1_line_b/1 -> [I1_line_b]
  Add1/1 -> Compare To Zero2/1
  [I1_line_b] -> Add1/1
  Add2/1 -> Compare To Zero3/1
  [I1_line_c] -> Add2/1
  Compare To Zero2/1 -> Logical Operator7/2
  Logical Operator7/1 -> Logical Operator3/2
  Compare To Zero1/1 -> Logical Operator7/1
  Compare To Zero3/1 -> Logical Operator7/3
  RNM_forward/1 -> [RNM_forward]
  RNM_reverse/1 -> [RNM_reverse]
  set_ena_dir/1 -> [set_ena_dir]
  set_dir/1 -> [set_dir]
  Logical Operator2/1 -> Logical Operator3/1
  [set_ena_dir] -> Logical Operator1/1
  Logical Operator1/1 -> Logical Operator2/3
  [RNM_forward] -> Logical Operator4/1
  [RNM_reverse] -> Logical Operator8/1
  [set_dir] -> Logical Operator4/2, Logical Operator9/1
  Logical Operator9/1 -> Logical Operator8/2
  Logical Operator8/1 -> Logical Operator2/2
  Logical Operator4/1 -> Logical Operator2/1
  Logical Operator3/1 -> start_AOPO1/1, [Start], relay_t/1(In)
  set_ena_step1/1 -> [set_ena_step1]
  set_ena_AOPO/1 -> [set_ena_AOPO]
  [set_ena_AOPO] -> Logical Operator3/4
  [set_ena_step1] -> Logical Operator3/5
  [set_tvv] -> relay_t/2(t_vv)
  [Block] -> Logical Operator6/2
  Logical Operator6/1 -> Logical Operator5/1
  [set_ena_dir] -> Logical Operator6/1
  Block_KTC/1 -> [Block_KTC]
  [Block_KTC] -> Logical Operator10/1
  Logical Operator10/1 -> Logical Operator3/6
  relay_t/1(Out) -> pulse_limited/1(In)
  pulse_limited/1(Out) -> trip_AOPO1/1
  Constant1/1 -> pulse_limited/2(t_pulse)

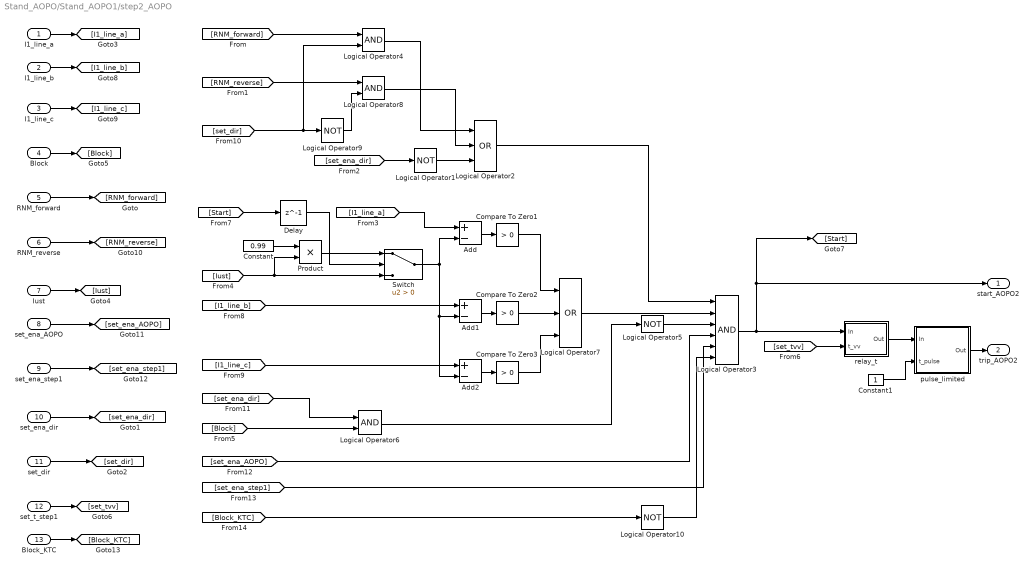
== system Stand_AOPO/Stand_AOPO1/step2_AOPO ==
  I1_line_a : Inport
  I1_line_b : Inport  Port=2
  I1_line_c : Inport  Port=3
  Block : Inport  Port=4
  RNM_forward : Inport  Port=5
  RNM_reverse : Inport  Port=6
  Iust : Inport  Port=7
  set_ena_AOPO : Inport  Port=8
  set_ena_step1 : Inport  Port=9
  set_ena_dir : Inport  Port=10
  set_dir : Inport  Port=11
  set_t_step1 : Inport  Port=12
  Block_KTC : Inport  Port=13
  Add : Sum  Inputs=+-
  Add1 : Sum  Inputs=+-
  Add2 : Sum  Inputs=+-
  Compare To Zero1 : simulink/Logic and Bit Operations/Compare To Zero  relop=>  OutDataTypeStr=boolean
  Compare To Zero2 : simulink/Logic and Bit Operations/Compare To Zero  relop=>  OutDataTypeStr=boolean
  Compare To Zero3 : simulink/Logic and Bit Operations/Compare To Zero  relop=>  OutDataTypeStr=boolean
  Constant : Constant  Value=0.99
  Constant1 : Constant
  Delay : Delay  DelayLength=1  InitialCondition=0
  Logical Operator{1,5,9..10} (4 alike) : Logic  Operator=NOT  AllPortsSameDT=off  OutDataTypeStr=boolean
  Logical Operator2 : Logic  Operator=OR  Inputs=3  AllPortsSameDT=off  OutDataTypeStr=boolean
  Logical Operator3 : Logic  Inputs=6  AllPortsSameDT=off  OutDataTypeStr=boolean
  Logical Operator4 : Logic  AllPortsSameDT=off  OutDataTypeStr=boolean
  Logical Operator6 : Logic  AllPortsSameDT=off  OutDataTypeStr=boolean
  Logical Operator7 : Logic  Operator=OR  Inputs=3  AllPortsSameDT=off  OutDataTypeStr=boolean
  Logical Operator8 : Logic  AllPortsSameDT=off  OutDataTypeStr=boolean
  Product : Product
  Switch : Switch  Criteria=u2 > Threshold
  pulse_limited : Subsystem
  relay_t : Subsystem
  start_AOPO2 : Outport
  trip_AOPO2 : Outport  Port=2
  wires:
  Constant1/1 -> pulse_limited/2(t_pulse)
  pulse_limited/1(Out) -> trip_AOPO2/1
  relay_t/1(Out) -> pulse_limited/1(In)
  Logical Operator10/1 -> Logical Operator3/6
  [Block_KTC] -> Logical Operator10/1
  Block_KTC/1 -> [Block_KTC]
  [set_ena_dir] -> Logical Operator6/1
  Logical Operator6/1 -> Logical Operator5/1
  [Block] -> Logical Operator6/2
  [set_tvv] -> relay_t/2(t_vv)
  [set_ena_step1] -> Logical Operator3/5
  [set_ena_AOPO] -> Logical Operator3/4
  set_ena_AOPO/1 -> [set_ena_AOPO]
  set_ena_step1/1 -> [set_ena_step1]
  Logical Operator3/1 -> relay_t/1(In), [Start], start_AOPO2/1
  Logical Operator4/1 -> Logical Operator2/1
  Logical Operator8/1 -> Logical Operator2/2
  Logical Operator9/1 -> Logical Operator8/2
  [set_dir] -> Logical Operator9/1, Logical Operator4/2
  [RNM_reverse] -> Logical Operator8/1
  [RNM_forward] -> Logical Operator4/1
  Logical Operator1/1 -> Logical Operator2/3
  [set_ena_dir] -> Logical Operator1/1
  Logical Operator2/1 -> Logical Operator3/1
  set_dir/1 -> [set_dir]
  set_ena_dir/1 -> [set_ena_dir]
  RNM_reverse/1 -> [RNM_reverse]
  RNM_forward/1 -> [RNM_forward]
  Compare To Zero3/1 -> Logical Operator7/3
  Compare To Zero1/1 -> Logical Operator7/1
  Logical Operator7/1 -> Logical Operator3/2
  Compare To Zero2/1 -> Logical Operator7/2
  [I1_line_c] -> Add2/1
  Add2/1 -> Compare To Zero3/1
  [I1_line_b] -> Add1/1
  Add1/1 -> Compare To Zero2/1
  I1_line_b/1 -> [I1_line_b]
  I1_line_c/1 -> [I1_line_c]
  Delay/1 -> Switch/2
  [Start] -> Delay/1
  Switch/1 -> Add/2, Add1/2, Add2/2
  Product/1 -> Switch/1
  Constant/1 -> Product/1
  [Iust] -> Product/2, Switch/3
  [I1_line_a] -> Add/1
  Add/1 -> Compare To Zero1/1
  Block/1 -> [Block]
  Iust/1 -> [Iust]
  set_t_step1/1 -> [set_tvv]
  Logical Operator5/1 -> Logical Operator3/3
  I1_line_a/1 -> [I1_line_a]

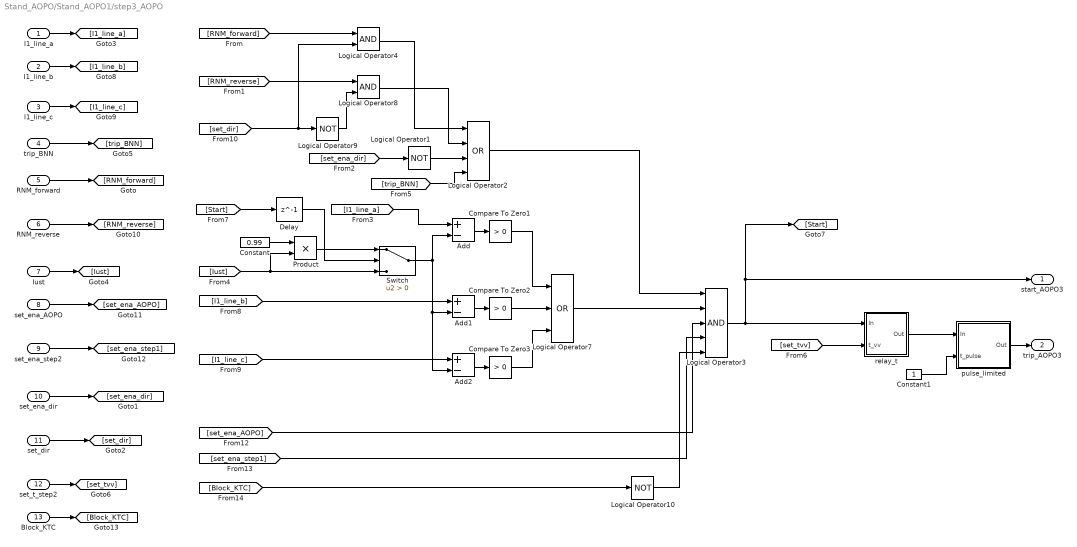
== system Stand_AOPO/Stand_AOPO1/step3_AOPO ==
  I1_line_a : Inport
  I1_line_b : Inport  Port=2
  I1_line_c : Inport  Port=3
  trip_BNN : Inport  Port=4
  RNM_forward : Inport  Port=5
  RNM_reverse : Inport  Port=6
  Iust : Inport  Port=7
  set_ena_AOPO : Inport  Port=8
  set_ena_step2 : Inport  Port=9
  set_ena_dir : Inport  Port=10
  set_dir : Inport  Port=11
  set_t_step2 : Inport  Port=12
  Block_KTC : Inport  Port=13
  Add : Sum  Inputs=+-
  Add1 : Sum  Inputs=+-
  Add2 : Sum  Inputs=+-
  Compare To Zero1 : simulink/Logic and Bit Operations/Compare To Zero  relop=>  OutDataTypeStr=boolean
  Compare To Zero2 : simulink/Logic and Bit Operations/Compare To Zero  relop=>  OutDataTypeStr=boolean
  Compare To Zero3 : simulink/Logic and Bit Operations/Compare To Zero  relop=>  OutDataTypeStr=boolean
  Constant : Constant  Value=0.99
  Constant1 : Constant
  Delay : Delay  DelayLength=1  InitialCondition=0
  Logical Operator1 : Logic  Operator=NOT  AllPortsSameDT=off  OutDataTypeStr=boolean
  Logical Operator10 : Logic  Operator=NOT  AllPortsSameDT=off  OutDataTypeStr=boolean
  Logical Operator2 : Logic  Operator=OR  Inputs=4  AllPortsSameDT=off  OutDataTypeStr=boolean
  Logical Operator3 : Logic  Inputs=5  AllPortsSameDT=off  OutDataTypeStr=boolean
  Logical Operator4 : Logic  AllPortsSameDT=off  OutDataTypeStr=boolean
  Logical Operator7 : Logic  Operator=OR  Inputs=3  AllPortsSameDT=off  OutDataTypeStr=boolean
  Logical Operator8 : Logic  AllPortsSameDT=off  OutDataTypeStr=boolean
  Logical Operator9 : Logic  Operator=NOT  AllPortsSameDT=off  OutDataTypeStr=boolean
  Product : Product
  Switch : Switch  Criteria=u2 > Threshold
  pulse_limited : Subsystem
  relay_t : Subsystem
  start_AOPO3 : Outport
  trip_AOPO3 : Outport  Port=2
  wires:
  [trip_BNN] -> Logical Operator2/4
  trip_BNN/1 -> [trip_BNN]
  pulse_limited/1(Out) -> trip_AOPO3/1
  relay_t/1(Out) -> pulse_limited/1(In)
  Constant1/1 -> pulse_limited/2(t_pulse)
  Logical Operator10/1 -> Logical Operator3/5
  [Block_KTC] -> Logical Operator10/1
  Block_KTC/1 -> [Block_KTC]
  [set_tvv] -> relay_t/2(t_vv)
  I1_line_a/1 -> [I1_line_a]
  set_t_step2/1 -> [set_tvv]
  Iust/1 -> [Iust]
  Add/1 -> Compare To Zero1/1
  [I1_line_a] -> Add/1
  [Iust] -> Switch/3, Product/2
  Constant/1 -> Product/1
  Product/1 -> Switch/1
  Switch/1 -> Add2/2, Add1/2, Add/2
  [Start] -> Delay/1
  Delay/1 -> Switch/2
  I1_line_c/1 -> [I1_line_c]
  I1_line_b/1 -> [I1_line_b]
  Add1/1 -> Compare To Zero2/1
  [I1_line_b] -> Add1/1
  Add2/1 -> Compare To Zero3/1
  [I1_line_c] -> Add2/1
  Compare To Zero2/1 -> Logical Operator7/2
  Logical Operator7/1 -> Logical Operator3/2
  Compare To Zero1/1 -> Logical Operator7/1
  Compare To Zero3/1 -> Logical Operator7/3
  RNM_forward/1 -> [RNM_forward]
  RNM_reverse/1 -> [RNM_reverse]
  set_ena_dir/1 -> [set_ena_dir]
  set_dir/1 -> [set_dir]
  Logical Operator2/1 -> Logical Operator3/1
  [set_ena_dir] -> Logical Operator1/1
  Logical Operator1/1 -> Logical Operator2/3
  [RNM_forward] -> Logical Operator4/1
  [RNM_reverse] -> Logical Operator8/1
  [set_dir] -> Logical Operator4/2, Logical Operator9/1
  Logical Operator9/1 -> Logical Operator8/2
  Logical Operator8/1 -> Logical Operator2/2
  Logical Operator4/1 -> Logical Operator2/1
  Logical Operator3/1 -> relay_t/1(In), start_AOPO3/1, [Start]
  set_ena_step2/1 -> [set_ena_step1]
  set_ena_AOPO/1 -> [set_ena_AOPO]
  [set_ena_AOPO] -> Logical Operator3/3
  [set_ena_step1] -> Logical Operator3/4

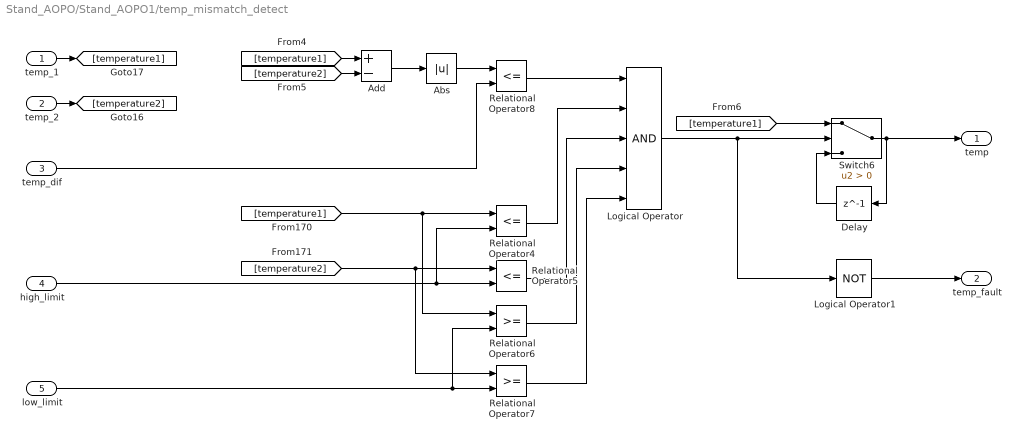
== system Stand_AOPO/Stand_AOPO1/temp_mismatch_detect ==
  temp_1 : Inport
  temp_2 : Inport  Port=2
  temp_dif : Inport  Port=3
  high_limit : Inport  Port=4
  low_limit : Inport  Port=5
  Abs : Abs
  Add : Sum  Inputs=+-
  Delay : Delay  DelayLength=1  InitialCondition=0
  Logical Operator : Logic  Inputs=5  AllPortsSameDT=off  OutDataTypeStr=boolean
  Logical Operator1 : Logic  Operator=NOT  Inputs=5  AllPortsSameDT=off  OutDataTypeStr=boolean
  Relational Operator4 : RelationalOperator  Operator=<=  OutDataTypeStr=boolean  RndMeth=Simplest
  Relational Operator5 : RelationalOperator  Operator=<=  OutDataTypeStr=boolean  RndMeth=Simplest
  Relational Operator6 : RelationalOperator  OutDataTypeStr=boolean  RndMeth=Simplest
  Relational Operator7 : RelationalOperator  OutDataTypeStr=boolean  RndMeth=Simplest
  Relational Operator8 : RelationalOperator  Operator=<=  OutDataTypeStr=boolean  RndMeth=Simplest
  Switch6 : Switch  Criteria=u2 > Threshold
  temp : Outport
  temp_fault : Outport  Port=2
  wires:
  Relational Operator4/1 -> Logical Operator/2
  [temperature2] -> Add/2
  [temperature1] -> Add/1
  Add/1 -> Abs/1
  Switch6/1 -> temp/1, Delay/1
  low_limit/1 -> Relational Operator6/2, Relational Operator7/2
  Relational Operator7/1 -> Logical Operator/5
  Relational Operator8/1 -> Logical Operator/1
  high_limit/1 -> Relational Operator5/2, Relational Operator4/2
  [temperature2] -> Relational Operator7/1, Relational Operator5/1
  Logical Operator/1 -> Logical Operator1/1, Switch6/2
  Abs/1 -> Relational Operator8/1
  Delay/1 -> Switch6/3
  [temperature1] -> Relational Operator6/1, Relational Operator4/1
  Relational Operator5/1 -> Logical Operator/3
  Relational Operator6/1 -> Logical Operator/4
  temp_dif/1 -> Relational Operator8/2
  [temperature1] -> Switch6/1
  temp_1/1 -> [temperature1]
  temp_2/1 -> [temperature2]
  Logical Operator1/1 -> temp_fault/1

== system Stand_AOPO/Stand_AOPO1/BNN/relay_t ==
  In : Inport
  t_vv : Inport  Port=2
  Data Type Conversion : DataTypeConversion  OutDataTypeStr=double
  Integrator1 : Integrator  ExternalReset=rising  LimitOutput=on  UpperSaturationLimit=10000
  Logical Operator2 : Logic  Operator=NOT  AllPortsSameDT=off  OutDataTypeStr=boolean
  Relational Operator : RelationalOperator  Operator=>  OutDataTypeStr=boolean  RndMeth=Nearest
  Out : Outport
  wires:
  Logical Operator2/1 -> Integrator1/2
  In/1 -> Data Type Conversion/1, Logical Operator2/1
  Relational Operator/1 -> Out/1
  Integrator1/1 -> Relational Operator/1
  t_vv/1 -> Relational Operator/2
  Data Type Conversion/1 -> Integrator1/1

== system Stand_AOPO/Stand_AOPO1/KTC/relay_t ==
  In : Inport
  t_vv : Inport  Port=2
  Data Type Conversion : DataTypeConversion  OutDataTypeStr=double
  Integrator1 : Integrator  ExternalReset=rising  LimitOutput=on  UpperSaturationLimit=10000
  Logical Operator2 : Logic  Operator=NOT  AllPortsSameDT=off  OutDataTypeStr=boolean
  Relational Operator : RelationalOperator  Operator=>  OutDataTypeStr=boolean  RndMeth=Nearest
  Out : Outport
  wires:
  Logical Operator2/1 -> Integrator1/2
  In/1 -> Data Type Conversion/1, Logical Operator2/1
  Relational Operator/1 -> Out/1
  Integrator1/1 -> Relational Operator/1
  t_vv/1 -> Relational Operator/2
  Data Type Conversion/1 -> Integrator1/1

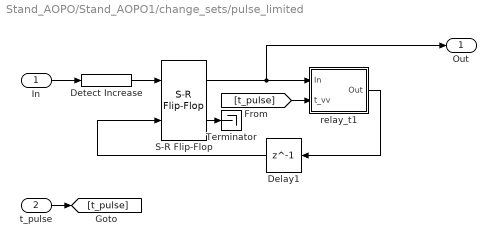
== system Stand_AOPO/Stand_AOPO1/change_sets/pulse_limited ==
  In : Inport
  t_pulse : Inport  Port=2
  Delay1 : Delay  DelayLength=1  InitialCondition=0
  Detect Increase : simulink/Logic and Bit Operations/Detect Increase  vinit=0.0  OutDataTypeStr=boolean
  S-R Flip-Flop : simulink_extras/Flip Flops/S-R Flip-Flop  initial_condition=0
  Terminator : Terminator
  relay_t1 : Subsystem
  Out : Outport
  wires:
  relay_t1/1(Out) -> Delay1/1
  S-R Flip-Flop/1 -> Out/1, relay_t1/1(In)
  Delay1/1 -> S-R Flip-Flop/2
  Detect Increase/1 -> S-R Flip-Flop/1
  [t_pulse] -> relay_t1/2(t_vv)
  In/1 -> Detect Increase/1
  S-R Flip-Flop/2 -> Terminator/1
  t_pulse/1 -> [t_pulse]

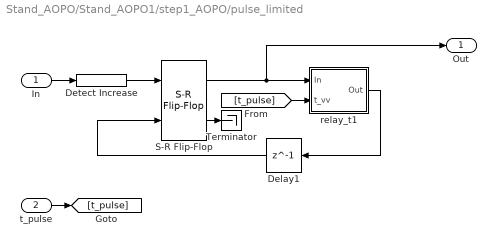
== system Stand_AOPO/Stand_AOPO1/step1_AOPO/pulse_limited ==
  In : Inport
  t_pulse : Inport  Port=2
  Delay1 : Delay  DelayLength=1  InitialCondition=0
  Detect Increase : simulink/Logic and Bit Operations/Detect Increase  vinit=0.0  OutDataTypeStr=boolean
  S-R Flip-Flop : simulink_extras/Flip Flops/S-R Flip-Flop  initial_condition=0
  Terminator : Terminator
  relay_t1 : Subsystem
  Out : Outport
  wires:
  relay_t1/1(Out) -> Delay1/1
  S-R Flip-Flop/1 -> Out/1, relay_t1/1(In)
  Delay1/1 -> S-R Flip-Flop/2
  Detect Increase/1 -> S-R Flip-Flop/1
  [t_pulse] -> relay_t1/2(t_vv)
  In/1 -> Detect Increase/1
  S-R Flip-Flop/2 -> Terminator/1
  t_pulse/1 -> [t_pulse]

== system Stand_AOPO/Stand_AOPO1/step1_AOPO/relay_t ==
  In : Inport
  t_vv : Inport  Port=2
  Data Type Conversion : DataTypeConversion  OutDataTypeStr=double
  Integrator1 : Integrator  ExternalReset=rising  LimitOutput=on  UpperSaturationLimit=10000
  Logical Operator2 : Logic  Operator=NOT  AllPortsSameDT=off  OutDataTypeStr=boolean
  Relational Operator : RelationalOperator  Operator=>  OutDataTypeStr=boolean  RndMeth=Nearest
  Out : Outport
  wires:
  Logical Operator2/1 -> Integrator1/2
  In/1 -> Data Type Conversion/1, Logical Operator2/1
  Relational Operator/1 -> Out/1
  Integrator1/1 -> Relational Operator/1
  t_vv/1 -> Relational Operator/2
  Data Type Conversion/1 -> Integrator1/1

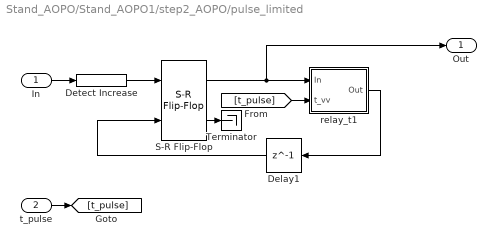
== system Stand_AOPO/Stand_AOPO1/step2_AOPO/pulse_limited ==
  In : Inport
  t_pulse : Inport  Port=2
  Delay1 : Delay  DelayLength=1  InitialCondition=0
  Detect Increase : simulink/Logic and Bit Operations/Detect Increase  vinit=0.0  OutDataTypeStr=boolean
  S-R Flip-Flop : simulink_extras/Flip Flops/S-R Flip-Flop  initial_condition=0
  Terminator : Terminator
  relay_t1 : Subsystem
  Out : Outport
  wires:
  t_pulse/1 -> [t_pulse]
  S-R Flip-Flop/2 -> Terminator/1
  In/1 -> Detect Increase/1
  [t_pulse] -> relay_t1/2(t_vv)
  Detect Increase/1 -> S-R Flip-Flop/1
  Delay1/1 -> S-R Flip-Flop/2
  S-R Flip-Flop/1 -> relay_t1/1(In), Out/1
  relay_t1/1(Out) -> Delay1/1

== system Stand_AOPO/Stand_AOPO1/step2_AOPO/relay_t ==
  In : Inport
  t_vv : Inport  Port=2
  Data Type Conversion : DataTypeConversion  OutDataTypeStr=double
  Integrator1 : Integrator  ExternalReset=rising  LimitOutput=on  UpperSaturationLimit=10000
  Logical Operator2 : Logic  Operator=NOT  AllPortsSameDT=off  OutDataTypeStr=boolean
  Relational Operator : RelationalOperator  Operator=>  OutDataTypeStr=boolean  RndMeth=Nearest
  Out : Outport
  wires:
  Data Type Conversion/1 -> Integrator1/1
  t_vv/1 -> Relational Operator/2
  Integrator1/1 -> Relational Operator/1
  Relational Operator/1 -> Out/1
  In/1 -> Logical Operator2/1, Data Type Conversion/1
  Logical Operator2/1 -> Integrator1/2

== system Stand_AOPO/Stand_AOPO1/step3_AOPO/pulse_limited ==
  In : Inport
  t_pulse : Inport  Port=2
  Delay1 : Delay  DelayLength=1  InitialCondition=0
  Detect Increase : simulink/Logic and Bit Operations/Detect Increase  vinit=0.0  OutDataTypeStr=boolean
  S-R Flip-Flop : simulink_extras/Flip Flops/S-R Flip-Flop  initial_condition=0
  Terminator : Terminator
  relay_t1 : Subsystem
  Out : Outport
  wires:
  t_pulse/1 -> [t_pulse]
  S-R Flip-Flop/2 -> Terminator/1
  In/1 -> Detect Increase/1
  [t_pulse] -> relay_t1/2(t_vv)
  Detect Increase/1 -> S-R Flip-Flop/1
  Delay1/1 -> S-R Flip-Flop/2
  S-R Flip-Flop/1 -> relay_t1/1(In), Out/1
  relay_t1/1(Out) -> Delay1/1

== system Stand_AOPO/Stand_AOPO1/step3_AOPO/relay_t ==
  In : Inport
  t_vv : Inport  Port=2
  Data Type Conversion : DataTypeConversion  OutDataTypeStr=double
  Integrator1 : Integrator  ExternalReset=rising  LimitOutput=on  UpperSaturationLimit=10000
  Logical Operator2 : Logic  Operator=NOT  AllPortsSameDT=off  OutDataTypeStr=boolean
  Relational Operator : RelationalOperator  Operator=>  OutDataTypeStr=boolean  RndMeth=Nearest
  Out : Outport
  wires:
  Data Type Conversion/1 -> Integrator1/1
  t_vv/1 -> Relational Operator/2
  Integrator1/1 -> Relational Operator/1
  Relational Operator/1 -> Out/1
  In/1 -> Logical Operator2/1, Data Type Conversion/1
  Logical Operator2/1 -> Integrator1/2

== system Stand_AOPO/Stand_AOPO1/change_sets/pulse_limited/relay_t1 ==
  In : Inport
  t_vv : Inport  Port=2
  Data Type Conversion : DataTypeConversion  OutDataTypeStr=double
  Integrator1 : Integrator  ExternalReset=rising  LimitOutput=on  UpperSaturationLimit=10000
  Logical Operator2 : Logic  Operator=NOT  AllPortsSameDT=off  OutDataTypeStr=boolean
  Relational Operator : RelationalOperator  Operator=>  OutDataTypeStr=boolean  RndMeth=Nearest
  Out : Outport
  wires:
  Data Type Conversion/1 -> Integrator1/1
  t_vv/1 -> Relational Operator/2
  Integrator1/1 -> Relational Operator/1
  Relational Operator/1 -> Out/1
  In/1 -> Logical Operator2/1, Data Type Conversion/1
  Logical Operator2/1 -> Integrator1/2

== system Stand_AOPO/Stand_AOPO1/step1_AOPO/pulse_limited/relay_t1 ==
  In : Inport
  t_vv : Inport  Port=2
  Data Type Conversion : DataTypeConversion  OutDataTypeStr=double
  Integrator1 : Integrator  ExternalReset=rising  LimitOutput=on  UpperSaturationLimit=10000
  Logical Operator2 : Logic  Operator=NOT  AllPortsSameDT=off  OutDataTypeStr=boolean
  Relational Operator : RelationalOperator  Operator=>  OutDataTypeStr=boolean  RndMeth=Nearest
  Out : Outport
  wires:
  Data Type Conversion/1 -> Integrator1/1
  t_vv/1 -> Relational Operator/2
  Integrator1/1 -> Relational Operator/1
  Relational Operator/1 -> Out/1
  In/1 -> Logical Operator2/1, Data Type Conversion/1
  Logical Operator2/1 -> Integrator1/2

== system Stand_AOPO/Stand_AOPO1/step2_AOPO/pulse_limited/relay_t1 ==
  In : Inport
  t_vv : Inport  Port=2
  Data Type Conversion : DataTypeConversion  OutDataTypeStr=double
  Integrator1 : Integrator  ExternalReset=rising  LimitOutput=on  UpperSaturationLimit=10000
  Logical Operator2 : Logic  Operator=NOT  AllPortsSameDT=off  OutDataTypeStr=boolean
  Relational Operator : RelationalOperator  Operator=>  OutDataTypeStr=boolean  RndMeth=Nearest
  Out : Outport
  wires:
  Logical Operator2/1 -> Integrator1/2
  In/1 -> Data Type Conversion/1, Logical Operator2/1
  Relational Operator/1 -> Out/1
  Integrator1/1 -> Relational Operator/1
  t_vv/1 -> Relational Operator/2
  Data Type Conversion/1 -> Integrator1/1

== system Stand_AOPO/Stand_AOPO1/step3_AOPO/pulse_limited/relay_t1 ==
  In : Inport
  t_vv : Inport  Port=2
  Data Type Conversion : DataTypeConversion  OutDataTypeStr=double
  Integrator1 : Integrator  ExternalReset=rising  LimitOutput=on  UpperSaturationLimit=10000
  Logical Operator2 : Logic  Operator=NOT  AllPortsSameDT=off  OutDataTypeStr=boolean
  Relational Operator : RelationalOperator  Operator=>  OutDataTypeStr=boolean  RndMeth=Nearest
  Out : Outport
  wires:
  Logical Operator2/1 -> Integrator1/2
  In/1 -> Data Type Conversion/1, Logical Operator2/1
  Relational Operator/1 -> Out/1
  Integrator1/1 -> Relational Operator/1
  t_vv/1 -> Relational Operator/2
  Data Type Conversion/1 -> Integrator1/1
